simulink subsystem "full_model_robot_rigid"  (R2022a)
settings: Solver=VariableStepAuto  StartTime=0.0  StopTime=10.0  RelTol=1e-3
undefined symbols (not defined in the file): hFriction
settings Model: Creator=Philipp  LastModifiedBy=Philipp
settings DebuggingCC: UnconnectedInputMsg=warning  UnconnectedOutputMsg=warning  UnconnectedLineMsg=warning
settings RTWCC: DLArmComputeVersion=19.05

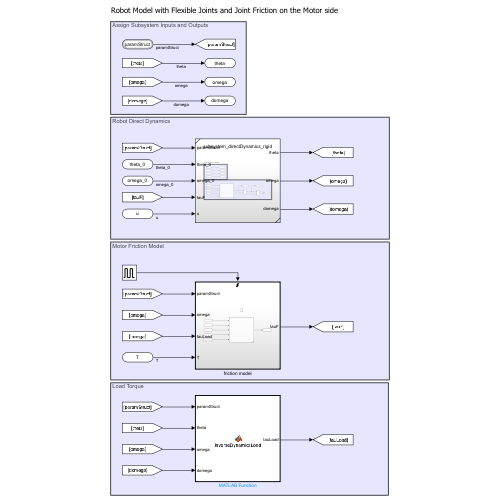
[thumbnail: Simulink's stored preview of the top-level diagram]
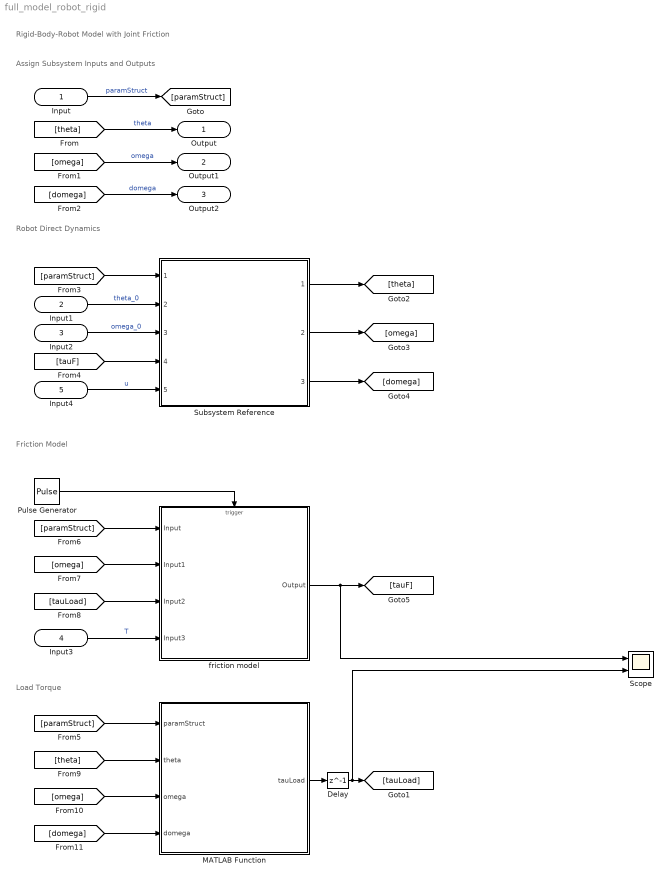
== system full_model_robot_rigid ==
  note: Load Torque
  note: Rigid-Body-Robot Model with Joint Friction
  note: Friction Model
  note: Robot Direct Dynamics
  note: Assign Subsystem Inputs and Outputs
  Input : Inport  OutDataTypeStr=Bus: main_bus
  Input1 : Inport  Port=2
  Input2 : Inport  Port=3
  Input3 : Inport  Port=4
  Input4 : Inport  Port=5  PortDimensions=3
  Delay : Delay  DelayLength=1  SampleTime=1e-3
  MATLAB Function : MATLAB Function  TreatAsAtomicUnit=on
  Pulse Generator : DiscretePulseGenerator  PulseType=Time based  Period=hFriction  PulseWidth=5
  Scope : Scope  NumInputPorts=2
  Subsystem Reference : Subsystem  ReferencedSubsystem=subsystem_directDynamics_rigid
  friction model : Subsystem  TreatAsAtomicUnit=on
  Output : Outport
  Output1 : Outport  Port=2
  Output2 : Outport  Port=3
  wires:
  Input/1 -> [paramStruct]  "paramStruct"
  [theta] -> Output/1  "theta"
  [domega] -> Output2/1  "domega"
  [omega] -> Output1/1  "omega"
  Input1/1 -> Subsystem Reference/2  "theta_0"
  [paramStruct] -> Subsystem Reference/1
  Input2/1 -> Subsystem Reference/3  "omega_0"
  Subsystem Reference/1 -> [theta]
  Subsystem Reference/3 -> [domega]
  Subsystem Reference/2 -> [omega]
  Pulse Generator/1 -> friction model/Trigger
  [paramStruct] -> friction model/1(Input)
  [omega] -> friction model/2(Input1)
  [tauLoad] -> friction model/3(Input2)
  Input3/1 -> friction model/4(Input3)  "T"
  friction model/1(Output) -> [tauF], Scope/1
  [tauF] -> Subsystem Reference/4
  Input4/1 -> Subsystem Reference/5  "u"
  [paramStruct] -> MATLAB Function/1(paramStruct)
  [theta] -> MATLAB Function/2(theta)
  [omega] -> MATLAB Function/3(omega)
  [domega] -> MATLAB Function/4(domega)
  MATLAB Function/1(tauLoad) -> Delay/1
  Delay/1 -> [tauLoad], Scope/2

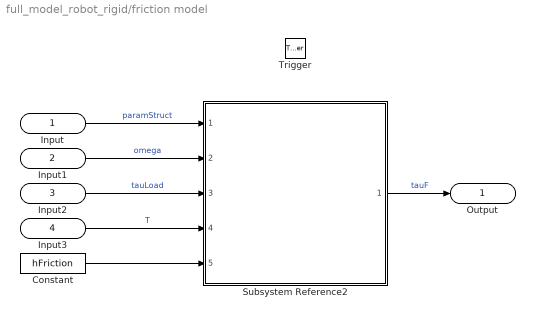
== system full_model_robot_rigid/friction model ==
  Input : Inport  OutDataTypeStr=Bus: main_bus
  Input1 : Inport  Port=2
  Input2 : Inport  Port=3
  Input3 : Inport  Port=4
  Trigger : TriggerPort  VariantControl=(inherit)
  Constant : Constant  Value=hFriction
  Subsystem Reference2 : Subsystem  ReferencedSubsystem=subsystem_lugreFriction
  Output : Outport  PortDimensions=3
  wires:
  Input3/1 -> Subsystem Reference2/4  "T"
  Input2/1 -> Subsystem Reference2/3  "tauLoad"
  Input1/1 -> Subsystem Reference2/2  "omega"
  Input/1 -> Subsystem Reference2/1  "paramStruct"
  Subsystem Reference2/1 -> Output/1  "tauF"
  Constant/1 -> Subsystem Reference2/5

== matlab function full_model_robot_rigid/MATLAB Function ==
  data: paramStruct input; tauLoad output; theta input; omega input; domega input
function tauLoad = inverseDynamicsLoad(paramStruct, theta, omega, domega)

g = paramStruct.robot.g;
r_P1P2 = paramStruct.robot.r_P1P2;
r_P2P3 = paramStruct.robot.r_P2P3;
r_P3P4 = paramStruct.robot.r_P3P4;
baseParam = paramStruct.robot.baseParam;

tauLoad = inverseDynamics_rigid_fun(g, r_P1P2, r_P2P3, r_P3P4, baseParam, theta, omega, domega, zeros(3,1));
